simulink model "sampleModel1782_1"  (R2023a)
settings: Solver=VariableStepAuto  StartTime=0.0  StopTime=10.0  RelTol=1e-3
libraries: hdlsllib x4
settings Model: Creator=user1  LastModifiedBy=user1

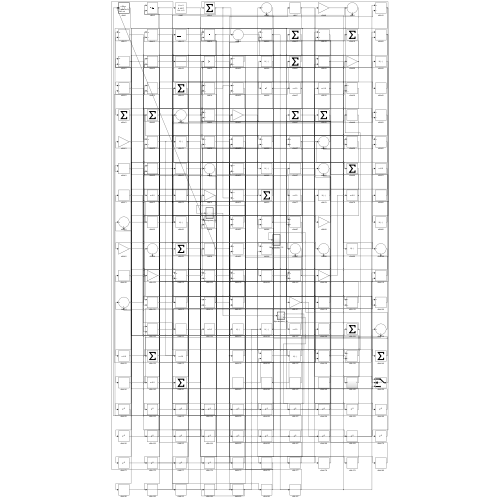
[thumbnail: Simulink's stored preview of the top-level diagram]
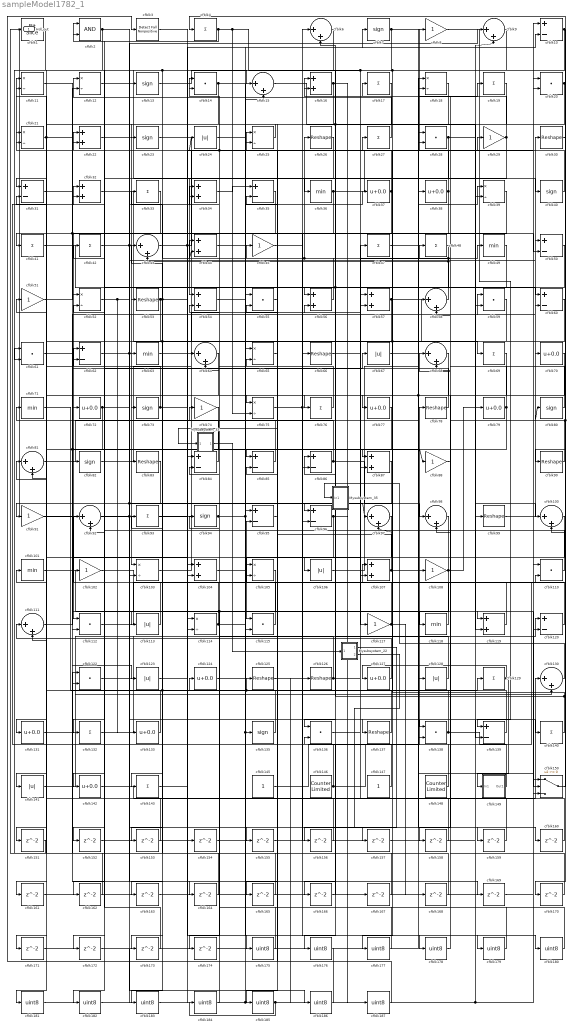
== system sampleModel1782_1 ==
  Mysubsystem_22 : Subsystem  TreatAsAtomicUnit=on  RTWFcnName=Mysubsystem_22
      settings: RTWFcnNameOpts=User specified  RTWFileNameOpts=Use function name
  Mysubsystem_33 : Subsystem  TreatAsAtomicUnit=on  RTWFcnName=Mysubsystem_33
      settings: RTWFcnNameOpts=User specified  RTWFileNameOpts=Use function name
  Mysubsystem_35 : Subsystem  TreatAsAtomicUnit=on  RTWFcnName=Mysubsystem_35
      settings: RTWFcnNameOpts=User specified  RTWFileNameOpts=Use function name
  cfblk1 : hdlsllib/Logic and Bit Operations/Bit Slice  lidx=7  ridx=0
  cfblk{10,31,35,50,60,62,84..86,95..96,120,139} (13 alike) : Sum  Inputs=+-  OutDataTypeStr=uint8
  cfblk{6,9,15,43,58,64,68,81,92,97..98,100,111,130} (14 alike) : Sum  Inputs=|++  OutDataTypeStr=uint8
  cfblk{36,49,63,71,101,118} (6 alike) : MinMax  OutDataTypeStr=uint8
  cfblk{8,29,45,51,74,88,91,102,108,117} (10 alike) : Gain  OutDataTypeStr=uint8
  cfblk{11..12,18,21,25,39,52,65,75,103,105,114} (12 alike) : Product  Inputs=*/  OutDataTypeStr=uint8  RndMeth=Zero  SaturateOnIntegerOverflow=on
  cfblk{16,22,32,34,44,54,56..57,87,104,107,119} (12 alike) : Sum  OutDataTypeStr=uint8
  cfblk{24,67,106,113,123,128,141} (7 alike) : Abs  OutDataTypeStr=uint8  SaturateOnIntegerOverflow=off
  cfblk{14,20,28,55,59,61,110,112,115,122,136,138} (12 alike) : DotProduct  OutDataTypeStr=uint8
  cfblk{37..38,70,72,77,79,124,127,131,133,142} (11 alike) : Bias  Bias=0.0  SaturateOnIntegerOverflow=off
  cfblk{26,30,53,66,78,83,90,99,125..126,137} (11 alike) : Reshape
  cfblk{4,17,19,27,33,41..42,47..48,69,76,93,129,132,140,143} (16 alike) : Sum  Inputs=+  OutDataTypeStr=uint8
  cfblk{7,13,23,40,73,80,82,94,135} (9 alike) : Signum
  cfblk145 : Constant  OutDataTypeStr=uint8  SampleTime=-1
  cfblk146 : hdlsllib/Sources/Counter Limited  uplimit=7  tsamp=-1
  cfblk147 : Constant  OutDataTypeStr=uint8  SampleTime=-1
  cfblk148 : hdlsllib/Sources/Counter Limited  uplimit=7  tsamp=-1
  cfblk149 : Subsystem
      settings: LibrarySourceBlock=|
      | hdlsllib/Ports &
      | Subsystems/Subsystem
  cfblk150 : Switch  OutDataTypeStr=uint8  SaturateOnIntegerOverflow=off  InputSameDT=off
  cfblk{151..174} (24 alike) : Delay  SampleTime=1
  cfblk{175..187} (13 alike) : DataTypeConversion  OutDataTypeStr=uint8  SaturateOnIntegerOverflow=off  RndMeth=Floor
  cfblk2 : Logic  AllPortsSameDT=off  OutDataTypeStr=boolean
  cfblk3 : hdlsllib/Logic and Bit Operations/Detect Fall Nonpositive  vinit=0  OutDataTypeStr=uint8
  Hdl_out : Outport  OutDataTypeStr=uint8
  wires:
  cfblk64/1 -> cfblk182/1
  cfblk23/1 -> cfblk69/1
  cfblk33/1 -> cfblk112/1
  cfblk65/1 -> cfblk185/1
  cfblk75/1 -> cfblk29/1, cfblk178/1
  cfblk7/1 -> cfblk54/1, cfblk59/2
  cfblk119/1 -> cfblk92/1
  cfblk8/1 -> cfblk139/1
  cfblk71/1 -> cfblk129/1
  cfblk58/1 -> cfblk26/1, cfblk25/2, cfblk43/2
  cfblk114/1 -> cfblk62/1, cfblk138/1
  cfblk41/1 -> cfblk56/1
  cfblk103/1 -> cfblk47/1
  cfblk38/1 -> cfblk8/1, cfblk86/2
  cfblk111/1 -> cfblk67/1
  cfblk20/1 -> cfblk103/1, cfblk100/2
  cfblk99/1 -> cfblk30/1
  cfblk148/1 -> cfblk32/1
  cfblk100/1 -> cfblk115/1
  cfblk73/1 -> cfblk51/1, cfblk118/1
  cfblk11/1 -> cfblk52/1
  cfblk146/1 -> cfblk45/1, cfblk128/1
  cfblk112/1 -> cfblk6/1
  cfblk137/1 -> cfblk93/1, cfblk21/2
  cfblk45/1 -> cfblk66/1
  cfblk107/1 -> cfblk35/2, cfblk160/1
  cfblk145/1 -> cfblk78/1
  cfblk49/1 -> cfblk96/1, cfblk132/1
  cfblk85/1 -> cfblk22/1
  cfblk74/1 -> cfblk113/1
  cfblk142/1 -> cfblk130/1
  cfblk118/1 -> cfblk95/2
  cfblk22/1 -> cfblk40/1
  cfblk27/1 -> cfblk12/1
  cfblk106/1 -> cfblk39/1
  cfblk59/1 -> cfblk83/1, cfblk181/1
  cfblk57/1 -> cfblk99/1, cfblk114/2
  cfblk60/1 -> cfblk115/2, cfblk77/1
  cfblk25/1 -> cfblk23/1
  cfblk37/1 -> cfblk136/1, cfblk16/1
  cfblk131/1 -> cfblk38/1
  cfblk32/1 -> cfblk105/1
  cfblk67/1 -> cfblk19/1
  cfblk53/1 -> cfblk84/1, cfblk143/1, cfblk131/1
  cfblk138/1 -> cfblk4/1, cfblk14/2
  cfblk101/1 -> cfblk150/1
  cfblk28/1 -> cfblk72/1, cfblk100/1
  cfblk125/1 -> cfblk137/1
  cfblk81/1 -> cfblk18/1
  cfblk123/1 -> cfblk28/1
  cfblk147/1 -> cfblk62/2
  cfblk82/1 -> cfblk56/2
  cfblk19/1 -> cfblk75/1
  cfblk48/1 -> cfblk76/1, cfblk44/2
  cfblk13/1 -> cfblk15/1
  cfblk34/1 -> cfblk35/1
  cfblk133/1 -> cfblk101/1
  cfblk140/1 -> cfblk27/1, cfblk86/1
  cfblk150/1 -> cfblk80/1, cfblk70/1
  cfblk80/1 -> cfblk17/1
  cfblk51/1 -> cfblk12/2
  cfblk84/1 -> cfblk71/1
  cfblk1/1 -> cfblk61/2
  cfblk30/1 -> cfblk90/1
  cfblk110/1 -> cfblk32/2
  cfblk92/1 -> cfblk9/1, cfblk104/2
  cfblk40/1 -> cfblk11/1
  cfblk139/1 -> cfblk74/1
  cfblk87/1 -> cfblk91/1
  cfblk42/1 -> cfblk105/2, cfblk87/2
  cfblk136/1 -> cfblk49/1
  cfblk6/1 -> cfblk31/1, cfblk163/1
  cfblk2/1 -> cfblk41/1, cfblk169/1
  cfblk31/1 -> cfblk50/2, cfblk164/1
  cfblk128/1 -> cfblk6/2
  cfblk10/1 -> cfblk57/2, cfblk36/1, cfblk170/1
  cfblk36/1 -> cfblk20/1, cfblk142/1
  cfblk4/1 -> cfblk117/1, cfblk75/2, cfblk2/2
  cfblk135/1 -> cfblk125/1, cfblk21/1
  cfblk9/1 -> cfblk97/2, cfblk152/1
  cfblk104/1 -> cfblk37/1
  cfblk132/1 -> cfblk120/1
  cfblk149/1(Out1) -> cfblk108/1
  cfblk105/1 -> cfblk122/2
  cfblk86/1 -> cfblk98/1, cfblk31/2
  cfblk43/1 -> cfblk25/1, cfblk10/2
  cfblk113/1 -> cfblk42/1
  cfblk21/1 -> cfblk88/1, cfblk103/2, cfblk171/1
  cfblk76/1 -> cfblk34/1
  cfblk90/1 -> cfblk48/1
  cfblk39/1 -> cfblk85/1
  cfblk52/1 -> cfblk13/1, cfblk133/1
  cfblk122/1 -> cfblk20/2
  cfblk26/1 -> cfblk73/1
  cfblk78/1 -> cfblk52/2
  cfblk54/1 -> cfblk135/1, cfblk179/1
  cfblk44/1 -> cfblk60/1
  cfblk108/1 -> cfblk174/1, cfblk183/1, cfblk106/1, cfblk79/1
  cfblk62/1 -> cfblk139/2, cfblk97/1, cfblk50/1
  cfblk17/1 -> cfblk82/1
  cfblk18/1 -> cfblk53/1, cfblk176/1
  cfblk143/1 -> cfblk107/1
  cfblk16/1 -> cfblk112/2, cfblk167/1
  cfblk66/1 -> cfblk120/2
  cfblk14/1 -> cfblk107/2, cfblk161/1
  cfblk102/1 -> cfblk119/1
  cfblk96/1 -> cfblk173/1, cfblk187/1
  cfblk72/1 -> cfblk34/2, cfblk81/2
  cfblk61/1 -> cfblk123/1
  cfblk126/1 -> cfblk94/1, cfblk110/2
  cfblk124/1 -> cfblk59/1
  cfblk15/1 -> cfblk119/2
  cfblk91/1 -> cfblk60/2
  cfblk141/1 -> cfblk130/2
  cfblk115/1 -> cfblk24/1, cfblk14/1
  cfblk29/1 -> cfblk16/2, cfblk166/1
  cfblk88/1 -> cfblk58/2
  cfblk94/1 -> cfblk7/1, cfblk140/1, Hdl_out/1
  cfblk56/1 -> cfblk33/1
  cfblk127/1 -> cfblk111/1
  cfblk117/1 -> cfblk2/1, cfblk168/1
  cfblk50/1 -> cfblk87/1
  cfblk79/1 -> cfblk44/1, cfblk102/1
  cfblk98/1 -> cfblk141/1
  cfblk70/1 -> cfblk111/2, cfblk138/2
  cfblk129/1 -> cfblk149/1(In1), cfblk127/1
  cfblk47/1 -> cfblk150/2
  cfblk120/1 -> cfblk98/2
  cfblk35/1 -> cfblk151/1
  cfblk151/1 -> cfblk1/1
  cfblk152/1 -> cfblk39/2
  cfblk97/1 -> cfblk153/1
  cfblk153/1 -> cfblk22/2
  cfblk93/1 -> cfblk154/1
  cfblk154/1 -> cfblk84/2
  cfblk12/1 -> cfblk155/1
  cfblk155/1 -> cfblk96/2
  cfblk156/1 -> cfblk85/2
  cfblk157/1 -> cfblk58/1
  cfblk69/1 -> cfblk158/1
  cfblk158/1 -> cfblk81/1
  cfblk24/1 -> cfblk159/1
  cfblk159/1 -> cfblk57/1
  cfblk160/1 -> cfblk54/2
  cfblk161/1 -> cfblk104/1
  cfblk77/1 -> cfblk162/1
  cfblk162/1 -> cfblk61/1
  cfblk163/1 -> cfblk10/1
  cfblk164/1 -> cfblk122/1
  cfblk55/1 -> cfblk165/1
  cfblk165/1 -> cfblk11/2
  cfblk166/1 -> cfblk136/2
  cfblk167/1 -> cfblk114/1
  cfblk168/1 -> cfblk43/1
  cfblk169/1 -> cfblk150/3
  cfblk170/1 -> cfblk18/2
  cfblk171/1 -> cfblk15/2
  cfblk83/1 -> cfblk172/1
  cfblk173/1 -> cfblk92/2
  cfblk174/1 -> cfblk28/2
  cfblk3/1 -> cfblk175/1
  cfblk175/1 -> cfblk124/1
  cfblk176/1 -> cfblk3/1
  cfblk68/1 -> cfblk177/1
  cfblk177/1 -> cfblk55/1
  cfblk178/1 -> cfblk68/1
  cfblk179/1 -> cfblk68/2
  cfblk63/1 -> cfblk180/1
  cfblk180/1 -> cfblk55/2
  cfblk181/1 -> cfblk63/1
  cfblk182/1 -> cfblk9/2, cfblk110/1, cfblk95/1
  cfblk183/1 -> cfblk64/1
  cfblk184/1 -> cfblk64/2
  cfblk185/1 -> cfblk184/1, cfblk126/1
  cfblk172/1 -> cfblk186/1
  cfblk186/1 -> cfblk65/1
  cfblk187/1 -> cfblk65/2
  Mysubsystem_22/1(Out1) -> cfblk156/1
  Mysubsystem_22/2(Out2) -> cfblk157/1
  cfblk95/1 -> Mysubsystem_33/1(In1)
  Mysubsystem_33/1(Out1) -> Mysubsystem_22/1(In1)
  cfblk130/1 -> Mysubsystem_35/1(In1)

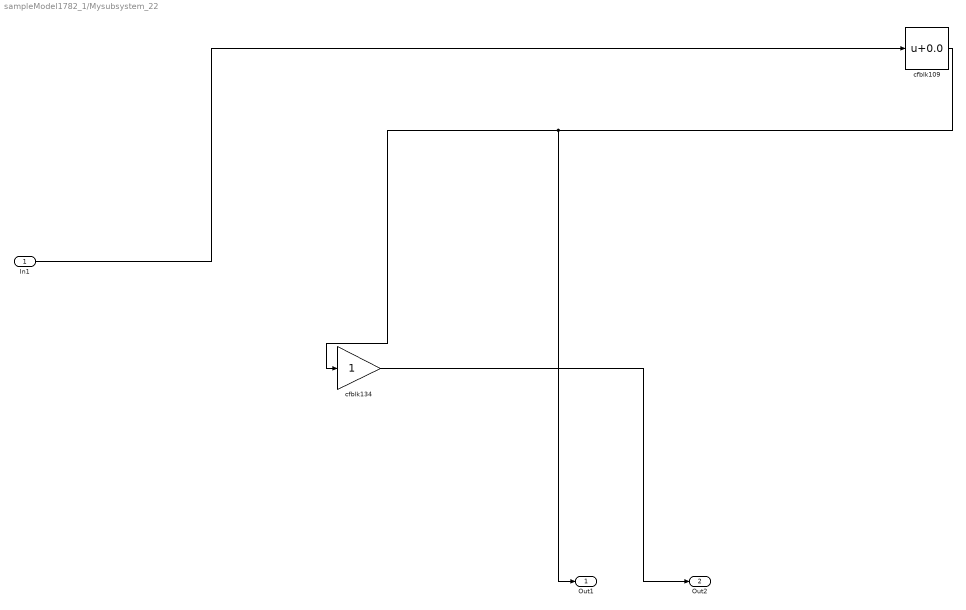
== system sampleModel1782_1/Mysubsystem_22 ==
  In1 : Inport
  cfblk109 : Bias  Bias=0.0  SaturateOnIntegerOverflow=off
  cfblk134 : Gain
  Out1 : Outport
  Out2 : Outport  Port=2
  wires:
  cfblk109/1 -> Out1/1, cfblk134/1
  cfblk134/1 -> Out2/1
  In1/1 -> cfblk109/1

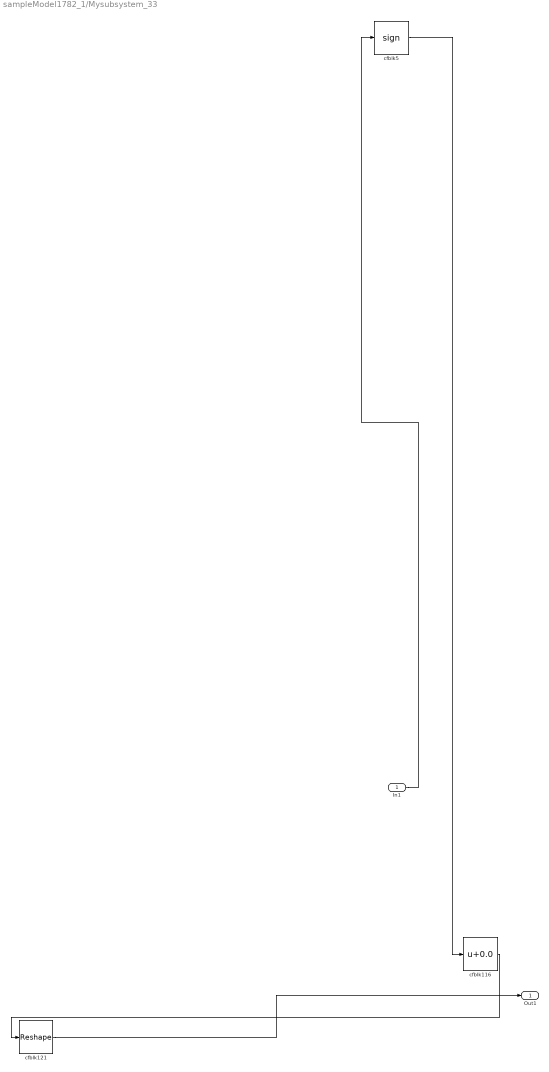
== system sampleModel1782_1/Mysubsystem_33 ==
  In1 : Inport
  cfblk116 : Bias  Bias=0.0  SaturateOnIntegerOverflow=off
  cfblk121 : Reshape
  cfblk5 : Signum
  Out1 : Outport
  wires:
  cfblk5/1 -> cfblk116/1
  cfblk116/1 -> cfblk121/1
  cfblk121/1 -> Out1/1
  In1/1 -> cfblk5/1

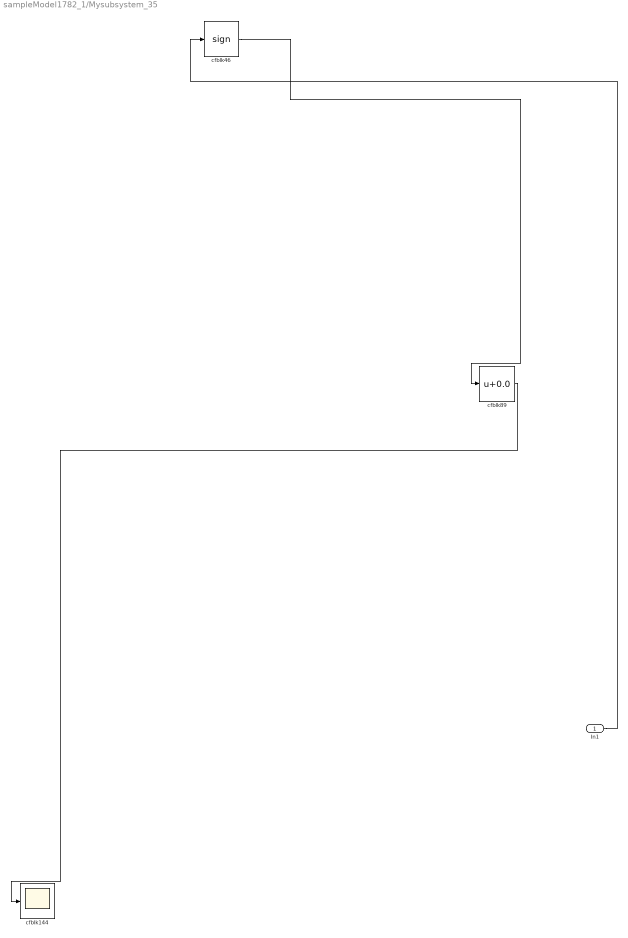
== system sampleModel1782_1/Mysubsystem_35 ==
  In1 : Inport
  cfblk144 : Scope
  cfblk46 : Signum
  cfblk89 : Bias  Bias=0.0  SaturateOnIntegerOverflow=off
  wires:
  cfblk89/1 -> cfblk144/1
  cfblk46/1 -> cfblk89/1
  In1/1 -> cfblk46/1

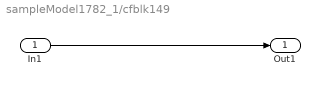
== system sampleModel1782_1/cfblk149 ==
  In1 : Inport
  Out1 : Outport
  wires:
  In1/1 -> Out1/1
